simulink model "c00007M_harness"  (R2018a)
settings: Solver=ode3  StartTime=0.0  StopTime=10.0  RelTol=1e-3  EnableMultiTasking=on
undefined symbols (not defined in the file): b, DiscIntNeverNeededParam, J, K, L, PosMinimaW3, PosMinimaW4, R, sigbuilder_block
(part 13 of 74)

== system c00007M_harness/M171 ==
  DW1 : Inport  OutMin=0  OutMax=4  OutDataTypeStr=int8
  DW2 : Inport  Port=2  OutMin=0  OutMax=4  OutDataTypeStr=int8
  DW3 : Inport  Port=3  OutMin=0  OutMax=4  OutDataTypeStr=int8
  P1W2 : Inport  Port=4  OutMin=0  OutMax=4  OutDataTypeStr=int8
  P2W3 : Inport  Port=5  OutMin=0  OutMax=4  OutDataTypeStr=int8
  P3W4 : Inport  Port=6  OutMin=0  OutMax=4  OutDataTypeStr=int8
  O1 : Inport  Port=7  OutDataTypeStr=boolean
  O2 : Inport  Port=8  OutDataTypeStr=boolean
  O3 : Inport  Port=9  OutDataTypeStr=boolean
  O4 : Inport  Port=10  OutDataTypeStr=boolean
  LD : Inport  Port=11  OutDataTypeStr=boolean
  CW1C : Inport  Port=12  OutMin=0  OutMax=4  OutDataTypeStr=int8
  CW2C : Inport  Port=13  OutMin=0  OutMax=4  OutDataTypeStr=int8
  CW4C : Inport  Port=14  OutMin=0  OutMax=4  OutDataTypeStr=int8
  Cyber : Subsystem
  M{,1..3} (4 alike) : Memory
  Physical : Subsystem
  S1 : Subsystem
  S2 : Subsystem
  S3 : Subsystem
  S4 : Subsystem
  W1Pos : Outport
  W2Pos : Outport  Port=2
  W3Pos : Outport  Port=3
  W4Pos : Outport  Port=4
  wires:
  Cyber/4(W4) -> Physical/4(InW4)
  Physical/4(W4) -> S4/1(PhyMeasure), W4Pos/1
  DW2/1 -> Cyber/6(DW2)
  P3W4/1 -> Cyber/10(P3W4)
  S2/1(SensorOut) -> M1/1
  Physical/2(W2) -> S2/1(PhyMeasure), W2Pos/1
  DW1/1 -> Cyber/5(DW1)
  M/1 -> Cyber/1(PosW1)
  Physical/3(W3) -> S3/1(PhyMeasure), W3Pos/1
  M1/1 -> Cyber/2(PosW2)
  S4/1(SensorOut) -> M3/1
  DW3/1 -> Cyber/7(DW3)
  O3/1 -> Cyber/13(OW3)
  CW1C/1 -> Cyber/16(CW1C)
  P1W2/1 -> Cyber/8(P1W2)
  M2/1 -> Cyber/3(PosW3)
  Cyber/2(W2) -> Physical/2(InW2)
  Cyber/1(W1) -> Physical/1(InW1)
  O1/1 -> Cyber/11(OW1)
  LD/1 -> Cyber/15(LD)
  Cyber/3(W3) -> Physical/3(InW3)
  O2/1 -> Cyber/12(OW2)
  S3/1(SensorOut) -> M2/1
  O4/1 -> Cyber/14(OW4)
  Physical/1(W1) -> S1/1(PhyMeasure), W1Pos/1
  CW4C/1 -> Cyber/18(CW4C)
  CW2C/1 -> Cyber/17(CW2C)
  S1/1(SensorOut) -> M/1
  P2W3/1 -> Cyber/9(P2W3)
  M3/1 -> Cyber/4(PosW4)

== system c00007M_harness/M172 ==
  DW1 : Inport  OutMin=0  OutMax=4  OutDataTypeStr=int8
  DW2 : Inport  Port=2  OutMin=0  OutMax=4  OutDataTypeStr=int8
  DW3 : Inport  Port=3  OutMin=0  OutMax=4  OutDataTypeStr=int8
  P1W2 : Inport  Port=4  OutMin=0  OutMax=4  OutDataTypeStr=int8
  P2W3 : Inport  Port=5  OutMin=0  OutMax=4  OutDataTypeStr=int8
  P3W4 : Inport  Port=6  OutMin=0  OutMax=4  OutDataTypeStr=int8
  O1 : Inport  Port=7  OutDataTypeStr=boolean
  O2 : Inport  Port=8  OutDataTypeStr=boolean
  O3 : Inport  Port=9  OutDataTypeStr=boolean
  O4 : Inport  Port=10  OutDataTypeStr=boolean
  LD : Inport  Port=11  OutDataTypeStr=boolean
  CW1C : Inport  Port=12  OutMin=0  OutMax=4  OutDataTypeStr=int8
  CW2C : Inport  Port=13  OutMin=0  OutMax=4  OutDataTypeStr=int8
  CW4C : Inport  Port=14  OutMin=0  OutMax=4  OutDataTypeStr=int8
  Cyber : Subsystem
  M{,1..3} (4 alike) : Memory
  Physical : Subsystem
  S1 : Subsystem
  S2 : Subsystem
  S3 : Subsystem
  S4 : Subsystem
  W1Pos : Outport
  W2Pos : Outport  Port=2
  W3Pos : Outport  Port=3
  W4Pos : Outport  Port=4
  wires:
  Cyber/4(W4) -> Physical/4(InW4)
  Physical/4(W4) -> S4/1(PhyMeasure), W4Pos/1
  DW2/1 -> Cyber/6(DW2)
  P3W4/1 -> Cyber/10(P3W4)
  S2/1(SensorOut) -> M1/1
  Physical/2(W2) -> S2/1(PhyMeasure), W2Pos/1
  DW1/1 -> Cyber/5(DW1)
  M/1 -> Cyber/1(PosW1)
  Physical/3(W3) -> S3/1(PhyMeasure), W3Pos/1
  M1/1 -> Cyber/2(PosW2)
  S4/1(SensorOut) -> M3/1
  DW3/1 -> Cyber/7(DW3)
  O3/1 -> Cyber/13(OW3)
  CW1C/1 -> Cyber/16(CW1C)
  P1W2/1 -> Cyber/8(P1W2)
  M2/1 -> Cyber/3(PosW3)
  Cyber/2(W2) -> Physical/2(InW2)
  Cyber/1(W1) -> Physical/1(InW1)
  O1/1 -> Cyber/11(OW1)
  LD/1 -> Cyber/15(LD)
  Cyber/3(W3) -> Physical/3(InW3)
  O2/1 -> Cyber/12(OW2)
  S3/1(SensorOut) -> M2/1
  O4/1 -> Cyber/14(OW4)
  Physical/1(W1) -> S1/1(PhyMeasure), W1Pos/1
  CW4C/1 -> Cyber/18(CW4C)
  CW2C/1 -> Cyber/17(CW2C)
  S1/1(SensorOut) -> M/1
  P2W3/1 -> Cyber/9(P2W3)
  M3/1 -> Cyber/4(PosW4)

== system c00007M_harness/M173 ==
  DW1 : Inport  OutMin=0  OutMax=4  OutDataTypeStr=int8
  DW2 : Inport  Port=2  OutMin=0  OutMax=4  OutDataTypeStr=int8
  DW3 : Inport  Port=3  OutMin=0  OutMax=4  OutDataTypeStr=int8
  P1W2 : Inport  Port=4  OutMin=0  OutMax=4  OutDataTypeStr=int8
  P2W3 : Inport  Port=5  OutMin=0  OutMax=4  OutDataTypeStr=int8
  P3W4 : Inport  Port=6  OutMin=0  OutMax=4  OutDataTypeStr=int8
  O1 : Inport  Port=7  OutDataTypeStr=boolean
  O2 : Inport  Port=8  OutDataTypeStr=boolean
  O3 : Inport  Port=9  OutDataTypeStr=boolean
  O4 : Inport  Port=10  OutDataTypeStr=boolean
  LD : Inport  Port=11  OutDataTypeStr=boolean
  CW1C : Inport  Port=12  OutMin=0  OutMax=4  OutDataTypeStr=int8
  CW2C : Inport  Port=13  OutMin=0  OutMax=4  OutDataTypeStr=int8
  CW4C : Inport  Port=14  OutMin=0  OutMax=4  OutDataTypeStr=int8
  Cyber : Subsystem
  M{,1..3} (4 alike) : Memory
  Physical : Subsystem
  S1 : Subsystem
  S2 : Subsystem
  S3 : Subsystem
  S4 : Subsystem
  W1Pos : Outport
  W2Pos : Outport  Port=2
  W3Pos : Outport  Port=3
  W4Pos : Outport  Port=4
  wires:
  Cyber/4(W4) -> Physical/4(InW4)
  Physical/4(W4) -> S4/1(PhyMeasure), W4Pos/1
  DW2/1 -> Cyber/6(DW2)
  P3W4/1 -> Cyber/10(P3W4)
  S2/1(SensorOut) -> M1/1
  Physical/2(W2) -> S2/1(PhyMeasure), W2Pos/1
  DW1/1 -> Cyber/5(DW1)
  M/1 -> Cyber/1(PosW1)
  Physical/3(W3) -> S3/1(PhyMeasure), W3Pos/1
  M1/1 -> Cyber/2(PosW2)
  S4/1(SensorOut) -> M3/1
  DW3/1 -> Cyber/7(DW3)
  O3/1 -> Cyber/13(OW3)
  CW1C/1 -> Cyber/16(CW1C)
  P1W2/1 -> Cyber/8(P1W2)
  M2/1 -> Cyber/3(PosW3)
  Cyber/2(W2) -> Physical/2(InW2)
  Cyber/1(W1) -> Physical/1(InW1)
  O1/1 -> Cyber/11(OW1)
  LD/1 -> Cyber/15(LD)
  Cyber/3(W3) -> Physical/3(InW3)
  O2/1 -> Cyber/12(OW2)
  S3/1(SensorOut) -> M2/1
  O4/1 -> Cyber/14(OW4)
  Physical/1(W1) -> S1/1(PhyMeasure), W1Pos/1
  CW4C/1 -> Cyber/18(CW4C)
  CW2C/1 -> Cyber/17(CW2C)
  S1/1(SensorOut) -> M/1
  P2W3/1 -> Cyber/9(P2W3)
  M3/1 -> Cyber/4(PosW4)

== system c00007M_harness/M174 ==
  DW1 : Inport  OutMin=0  OutMax=4  OutDataTypeStr=int8
  DW2 : Inport  Port=2  OutMin=0  OutMax=4  OutDataTypeStr=int8
  DW3 : Inport  Port=3  OutMin=0  OutMax=4  OutDataTypeStr=int8
  P1W2 : Inport  Port=4  OutMin=0  OutMax=4  OutDataTypeStr=int8
  P2W3 : Inport  Port=5  OutMin=0  OutMax=4  OutDataTypeStr=int8
  P3W4 : Inport  Port=6  OutMin=0  OutMax=4  OutDataTypeStr=int8
  O1 : Inport  Port=7  OutDataTypeStr=boolean
  O2 : Inport  Port=8  OutDataTypeStr=boolean
  O3 : Inport  Port=9  OutDataTypeStr=boolean
  O4 : Inport  Port=10  OutDataTypeStr=boolean
  LD : Inport  Port=11  OutDataTypeStr=boolean
  CW1C : Inport  Port=12  OutMin=0  OutMax=4  OutDataTypeStr=int8
  CW2C : Inport  Port=13  OutMin=0  OutMax=4  OutDataTypeStr=int8
  CW4C : Inport  Port=14  OutMin=0  OutMax=4  OutDataTypeStr=int8
  Cyber : Subsystem
  M{,1..3} (4 alike) : Memory
  Physical : Subsystem
  S1 : Subsystem
  S2 : Subsystem
  S3 : Subsystem
  S4 : Subsystem
  W1Pos : Outport
  W2Pos : Outport  Port=2
  W3Pos : Outport  Port=3
  W4Pos : Outport  Port=4
  wires:
  Cyber/4(W4) -> Physical/4(InW4)
  Physical/4(W4) -> S4/1(PhyMeasure), W4Pos/1
  DW2/1 -> Cyber/6(DW2)
  P3W4/1 -> Cyber/10(P3W4)
  S2/1(SensorOut) -> M1/1
  Physical/2(W2) -> S2/1(PhyMeasure), W2Pos/1
  DW1/1 -> Cyber/5(DW1)
  M/1 -> Cyber/1(PosW1)
  Physical/3(W3) -> S3/1(PhyMeasure), W3Pos/1
  M1/1 -> Cyber/2(PosW2)
  S4/1(SensorOut) -> M3/1
  DW3/1 -> Cyber/7(DW3)
  O3/1 -> Cyber/13(OW3)
  CW1C/1 -> Cyber/16(CW1C)
  P1W2/1 -> Cyber/8(P1W2)
  M2/1 -> Cyber/3(PosW3)
  Cyber/2(W2) -> Physical/2(InW2)
  Cyber/1(W1) -> Physical/1(InW1)
  O1/1 -> Cyber/11(OW1)
  LD/1 -> Cyber/15(LD)
  Cyber/3(W3) -> Physical/3(InW3)
  O2/1 -> Cyber/12(OW2)
  S3/1(SensorOut) -> M2/1
  O4/1 -> Cyber/14(OW4)
  Physical/1(W1) -> S1/1(PhyMeasure), W1Pos/1
  CW4C/1 -> Cyber/18(CW4C)
  CW2C/1 -> Cyber/17(CW2C)
  S1/1(SensorOut) -> M/1
  P2W3/1 -> Cyber/9(P2W3)
  M3/1 -> Cyber/4(PosW4)

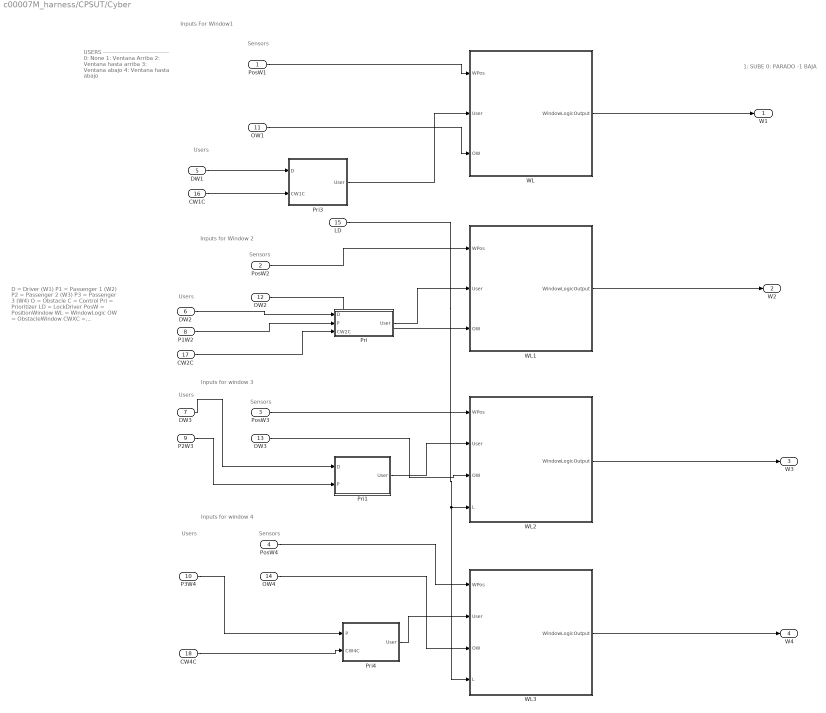
== system c00007M_harness/CPSUT/Cyber ==
  note: D = Driver (W1)
      | P1 = Passenger 1 (W2)
      | P2 = Passenger 2 (W3)
      | P3 = Passenger 3 (W4)
      | O = Obstacle
      | C = Control
      | Pri = Prioritizer
      | LD = LockDriver
      | PosW = PositionWindow
      | WL = WindowLogic
      | OW = ObstacleWindow
      | CWXC = ControlWindowXCentralized
      | S = Sensor
      | L = Lock
      | WPos = WindowPosition
      | M = Memory
      | InW = InputWindow
      | WIn = WindowInput
  note: 1: SUBE
      | 0: PARADO
      | -1 BAJA
  note: USERS
      | ---------------------------------
      | 0: None
      | 1: Ventana Arriba
      | 2: Ventana hasta arriba
      | 3: Ventana abajo
      | 4: Ventana hasta abajo
  note: Sensors
  note: Users
  note: Sensors
  note: Users
  note: Sensors
  note: Users
  note: Users
  note: Inputs for window 4
  note: Inputs for window 3
  note: Inputs for Window 2
  note: Inputs For Window1
  note: Sensors
  PosW1 : Inport
  PosW2 : Inport  Port=2
  PosW3 : Inport  Port=3
  PosW4 : Inport  Port=4
  DW1 : Inport  Port=5
  DW2 : Inport  Port=6
  DW3 : Inport  Port=7
  P1W2 : Inport  Port=8
  P2W3 : Inport  Port=9
  P3W4 : Inport  Port=10
  OW1 : Inport  Port=11
  OW2 : Inport  Port=12
  OW3 : Inport  Port=13
  OW4 : Inport  Port=14
  LD : Inport  Port=15
  CW1C : Inport  Port=16
  CW2C : Inport  Port=17
  CW4C : Inport  Port=18
  Pri : Subsystem
  Pri1 : Subsystem
  Pri3 : Subsystem
  Pri4 : Subsystem
  WL : Subsystem
  WL1 : Subsystem
  WL2 : Subsystem
  WL3 : Subsystem
  W1 : Outport
  W2 : Outport  Port=2
  W3 : Outport  Port=3
  W4 : Outport  Port=4
  wires:
  LD/1 -> WL3/4(L), WL2/4(L)
  PosW1/1 -> WL/1(WPos)
  OW1/1 -> WL/3(OW)
  DW1/1 -> Pri3/1(D)
  WL/1(WindowLogicOutput) -> W1/1
  Pri/1(User) -> WL1/2(User)
  DW2/1 -> Pri/1(D)
  P1W2/1 -> Pri/2(P)
  PosW2/1 -> WL1/1(WPos)
  OW2/1 -> WL1/3(OW)
  WL1/1(WindowLogicOutput) -> W2/1
  Pri1/1(User) -> WL2/2(User)
  PosW3/1 -> WL2/1(WPos)
  OW3/1 -> WL2/3(OW)
  DW3/1 -> Pri1/1(D)
  P2W3/1 -> Pri1/2(P)
  P3W4/1 -> Pri4/1(P)
  PosW4/1 -> WL3/1(WPos)
  OW4/1 -> WL3/3(OW)
  Pri4/1(User) -> WL3/2(User)
  WL2/1(WindowLogicOutput) -> W3/1
  WL3/1(WindowLogicOutput) -> W4/1
  Pri3/1(User) -> WL/2(User)
  CW1C/1 -> Pri3/2(CW1C)
  CW2C/1 -> Pri/3(CW2C)
  CW4C/1 -> Pri4/2(CW4C)

== system c00007M_harness/CPSUT/Physical ==
  InW1 : Inport
  InW2 : Inport  Port=2
  InW3 : Inport  Port=3
  InW4 : Inport  Port=4
  W : Subsystem
  W5 : Subsystem
  W6 : Subsystem
  W7 : Subsystem
  W1 : Outport
  W2 : Outport  Port=2
  W3 : Outport  Port=3
  W4 : Outport  Port=4
  wires:
  InW1/1 -> W/1(WIn)
  InW2/1 -> W5/1(WIn)
  InW3/1 -> W6/1(WIn)
  InW4/1 -> W7/1(WIn)
  W/1(WPos) -> W1/1
  W5/1(WPos) -> W2/1
  W6/1(WPos) -> W3/1
  W7/1(WPos) -> W4/1

== system c00007M_harness/CPSUT/S1 ==
  PhyMeasure : Inport
  SensorOut : Outport
  wires:
  PhyMeasure/1 -> SensorOut/1

== system c00007M_harness/CPSUT/S2 ==
  PhyMeasure : Inport
  SensorOut : Outport
  wires:
  PhyMeasure/1 -> SensorOut/1

== system c00007M_harness/CPSUT/S3 ==
  PhyMeasure : Inport
  SensorOut : Outport
  wires:
  PhyMeasure/1 -> SensorOut/1

== system c00007M_harness/CPSUT/S4 ==
  PhyMeasure : Inport
  SensorOut : Outport
  wires:
  PhyMeasure/1 -> SensorOut/1

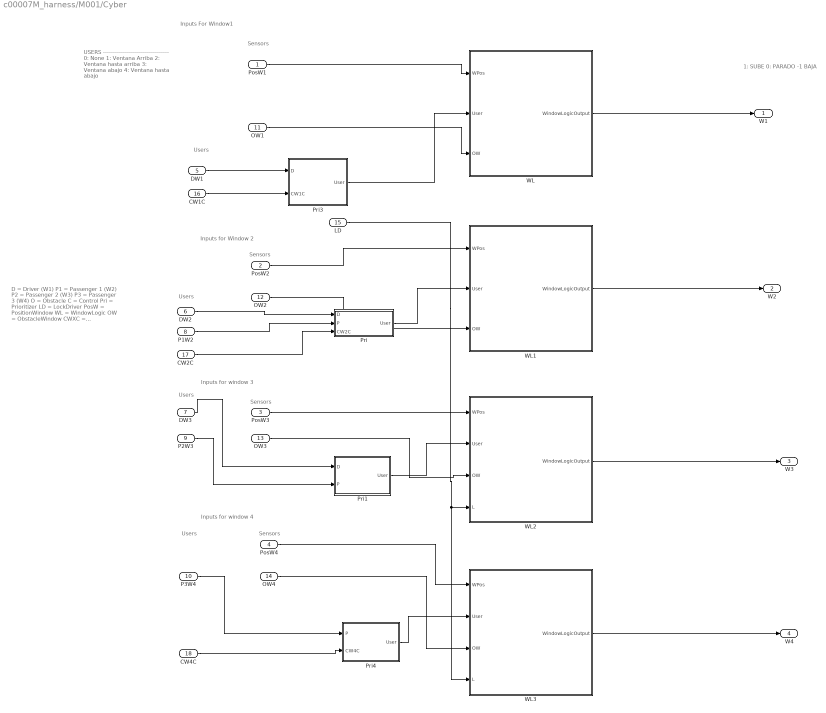
== system c00007M_harness/M001/Cyber ==
  note: D = Driver (W1)
      | P1 = Passenger 1 (W2)
      | P2 = Passenger 2 (W3)
      | P3 = Passenger 3 (W4)
      | O = Obstacle
      | C = Control
      | Pri = Prioritizer
      | LD = LockDriver
      | PosW = PositionWindow
      | WL = WindowLogic
      | OW = ObstacleWindow
      | CWXC = ControlWindowXCentralized
      | S = Sensor
      | L = Lock
      | WPos = WindowPosition
      | M = Memory
      | InW = InputWindow
      | WIn = WindowInput
  note: 1: SUBE
      | 0: PARADO
      | -1 BAJA
  note: USERS
      | ---------------------------------
      | 0: None
      | 1: Ventana Arriba
      | 2: Ventana hasta arriba
      | 3: Ventana abajo
      | 4: Ventana hasta abajo
  note: Sensors
  note: Users
  note: Sensors
  note: Users
  note: Sensors
  note: Users
  note: Users
  note: Inputs for window 4
  note: Inputs for window 3
  note: Inputs for Window 2
  note: Inputs For Window1
  note: Sensors
  PosW1 : Inport
  PosW2 : Inport  Port=2
  PosW3 : Inport  Port=3
  PosW4 : Inport  Port=4
  DW1 : Inport  Port=5
  DW2 : Inport  Port=6
  DW3 : Inport  Port=7
  P1W2 : Inport  Port=8
  P2W3 : Inport  Port=9
  P3W4 : Inport  Port=10
  OW1 : Inport  Port=11
  OW2 : Inport  Port=12
  OW3 : Inport  Port=13
  OW4 : Inport  Port=14
  LD : Inport  Port=15
  CW1C : Inport  Port=16
  CW2C : Inport  Port=17
  CW4C : Inport  Port=18
  Pri : Subsystem
  Pri1 : Subsystem
  Pri3 : Subsystem
  Pri4 : Subsystem
  WL : Subsystem
  WL1 : Subsystem
  WL2 : Subsystem
  WL3 : Subsystem
  W1 : Outport
  W2 : Outport  Port=2
  W3 : Outport  Port=3
  W4 : Outport  Port=4
  wires:
  LD/1 -> WL3/4(L), WL2/4(L)
  PosW1/1 -> WL/1(WPos)
  OW1/1 -> WL/3(OW)
  DW1/1 -> Pri3/1(D)
  WL/1(WindowLogicOutput) -> W1/1
  Pri/1(User) -> WL1/2(User)
  DW2/1 -> Pri/1(D)
  P1W2/1 -> Pri/2(P)
  PosW2/1 -> WL1/1(WPos)
  OW2/1 -> WL1/3(OW)
  WL1/1(WindowLogicOutput) -> W2/1
  Pri1/1(User) -> WL2/2(User)
  PosW3/1 -> WL2/1(WPos)
  OW3/1 -> WL2/3(OW)
  DW3/1 -> Pri1/1(D)
  P2W3/1 -> Pri1/2(P)
  P3W4/1 -> Pri4/1(P)
  PosW4/1 -> WL3/1(WPos)
  OW4/1 -> WL3/3(OW)
  Pri4/1(User) -> WL3/2(User)
  WL2/1(WindowLogicOutput) -> W3/1
  WL3/1(WindowLogicOutput) -> W4/1
  Pri3/1(User) -> WL/2(User)
  CW1C/1 -> Pri3/2(CW1C)
  CW2C/1 -> Pri/3(CW2C)
  CW4C/1 -> Pri4/2(CW4C)

== system c00007M_harness/M001/Physical ==
  InW1 : Inport
  InW2 : Inport  Port=2
  InW3 : Inport  Port=3
  InW4 : Inport  Port=4
  W : Subsystem
  W5 : Subsystem
  W6 : Subsystem
  W7 : Subsystem
  W1 : Outport
  W2 : Outport  Port=2
  W3 : Outport  Port=3
  W4 : Outport  Port=4
  wires:
  InW1/1 -> W/1(WIn)
  InW2/1 -> W5/1(WIn)
  InW3/1 -> W6/1(WIn)
  InW4/1 -> W7/1(WIn)
  W/1(WPos) -> W1/1
  W5/1(WPos) -> W2/1
  W6/1(WPos) -> W3/1
  W7/1(WPos) -> W4/1

== system c00007M_harness/M001/S1 ==
  PhyMeasure : Inport
  SensorOut : Outport
  wires:
  PhyMeasure/1 -> SensorOut/1

== system c00007M_harness/M001/S2 ==
  PhyMeasure : Inport
  SensorOut : Outport
  wires:
  PhyMeasure/1 -> SensorOut/1

== system c00007M_harness/M001/S3 ==
  PhyMeasure : Inport
  SensorOut : Outport
  wires:
  PhyMeasure/1 -> SensorOut/1

== system c00007M_harness/M001/S4 ==
  PhyMeasure : Inport
  SensorOut : Outport
  wires:
  PhyMeasure/1 -> SensorOut/1

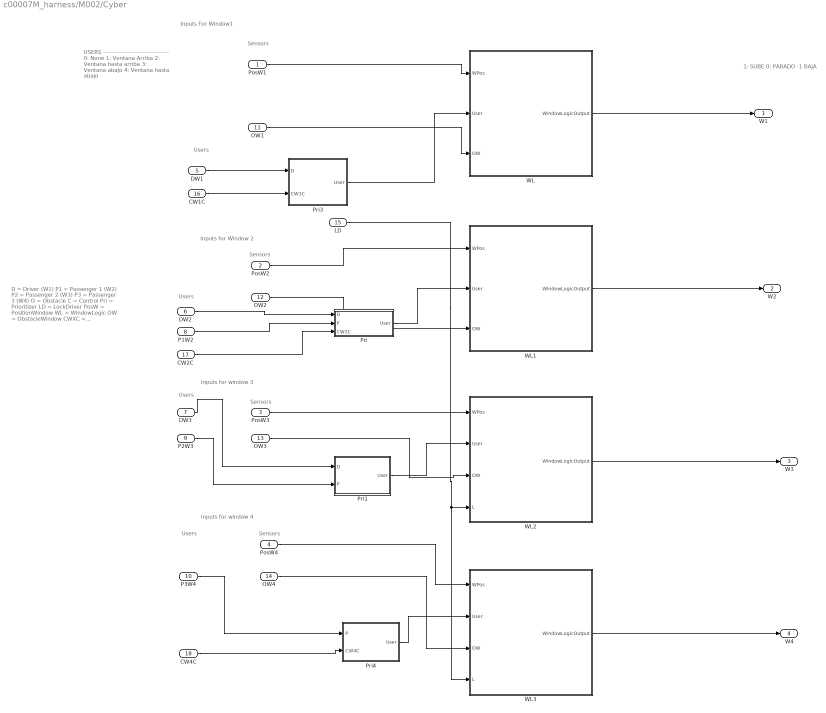
== system c00007M_harness/M002/Cyber ==
  note: Sensors
  note: Inputs For Window1
  note: Inputs for Window 2
  note: Inputs for window 3
  note: Inputs for window 4
  note: Users
  note: Users
  note: Sensors
  note: Users
  note: Sensors
  note: Users
  note: Sensors
  note: USERS
      | ---------------------------------
      | 0: None
      | 1: Ventana Arriba
      | 2: Ventana hasta arriba
      | 3: Ventana abajo
      | 4: Ventana hasta abajo
  note: 1: SUBE
      | 0: PARADO
      | -1 BAJA
  note: D = Driver (W1)
      | P1 = Passenger 1 (W2)
      | P2 = Passenger 2 (W3)
      | P3 = Passenger 3 (W4)
      | O = Obstacle
      | C = Control
      | Pri = Prioritizer
      | LD = LockDriver
      | PosW = PositionWindow
      | WL = WindowLogic
      | OW = ObstacleWindow
      | CWXC = ControlWindowXCentralized
      | S = Sensor
      | L = Lock
      | WPos = WindowPosition
      | M = Memory
      | InW = InputWindow
      | WIn = WindowInput
  PosW1 : Inport
  PosW2 : Inport  Port=2
  PosW3 : Inport  Port=3
  PosW4 : Inport  Port=4
  DW1 : Inport  Port=5
  DW2 : Inport  Port=6
  DW3 : Inport  Port=7
  P1W2 : Inport  Port=8
  P2W3 : Inport  Port=9
  P3W4 : Inport  Port=10
  OW1 : Inport  Port=11
  OW2 : Inport  Port=12
  OW3 : Inport  Port=13
  OW4 : Inport  Port=14
  LD : Inport  Port=15
  CW1C : Inport  Port=16
  CW2C : Inport  Port=17
  CW4C : Inport  Port=18
  Pri : Subsystem
  Pri1 : Subsystem
  Pri3 : Subsystem
  Pri4 : Subsystem
  WL : Subsystem
  WL1 : Subsystem
  WL2 : Subsystem
  WL3 : Subsystem
  W1 : Outport
  W2 : Outport  Port=2
  W3 : Outport  Port=3
  W4 : Outport  Port=4
  wires:
  CW4C/1 -> Pri4/2(CW4C)
  CW2C/1 -> Pri/3(CW2C)
  CW1C/1 -> Pri3/2(CW1C)
  Pri3/1(User) -> WL/2(User)
  WL3/1(WindowLogicOutput) -> W4/1
  WL2/1(WindowLogicOutput) -> W3/1
  Pri4/1(User) -> WL3/2(User)
  OW4/1 -> WL3/3(OW)
  PosW4/1 -> WL3/1(WPos)
  P3W4/1 -> Pri4/1(P)
  P2W3/1 -> Pri1/2(P)
  DW3/1 -> Pri1/1(D)
  OW3/1 -> WL2/3(OW)
  PosW3/1 -> WL2/1(WPos)
  Pri1/1(User) -> WL2/2(User)
  WL1/1(WindowLogicOutput) -> W2/1
  OW2/1 -> WL1/3(OW)
  PosW2/1 -> WL1/1(WPos)
  P1W2/1 -> Pri/2(P)
  DW2/1 -> Pri/1(D)
  Pri/1(User) -> WL1/2(User)
  WL/1(WindowLogicOutput) -> W1/1
  DW1/1 -> Pri3/1(D)
  OW1/1 -> WL/3(OW)
  PosW1/1 -> WL/1(WPos)
  LD/1 -> WL2/4(L), WL3/4(L)

== system c00007M_harness/M002/Physical ==
  InW1 : Inport
  InW2 : Inport  Port=2
  InW3 : Inport  Port=3
  InW4 : Inport  Port=4
  W : Subsystem
  W5 : Subsystem
  W6 : Subsystem
  W7 : Subsystem
  W1 : Outport
  W2 : Outport  Port=2
  W3 : Outport  Port=3
  W4 : Outport  Port=4
  wires:
  W7/1(WPos) -> W4/1
  W6/1(WPos) -> W3/1
  W5/1(WPos) -> W2/1
  W/1(WPos) -> W1/1
  InW4/1 -> W7/1(WIn)
  InW3/1 -> W6/1(WIn)
  InW2/1 -> W5/1(WIn)
  InW1/1 -> W/1(WIn)

== system c00007M_harness/M002/S1 ==
  PhyMeasure : Inport
  SensorOut : Outport
  wires:
  PhyMeasure/1 -> SensorOut/1

== system c00007M_harness/M002/S2 ==
  PhyMeasure : Inport
  SensorOut : Outport
  wires:
  PhyMeasure/1 -> SensorOut/1

== system c00007M_harness/M002/S3 ==
  PhyMeasure : Inport
  SensorOut : Outport
  wires:
  PhyMeasure/1 -> SensorOut/1

== system c00007M_harness/M002/S4 ==
  PhyMeasure : Inport
  SensorOut : Outport
  wires:
  PhyMeasure/1 -> SensorOut/1

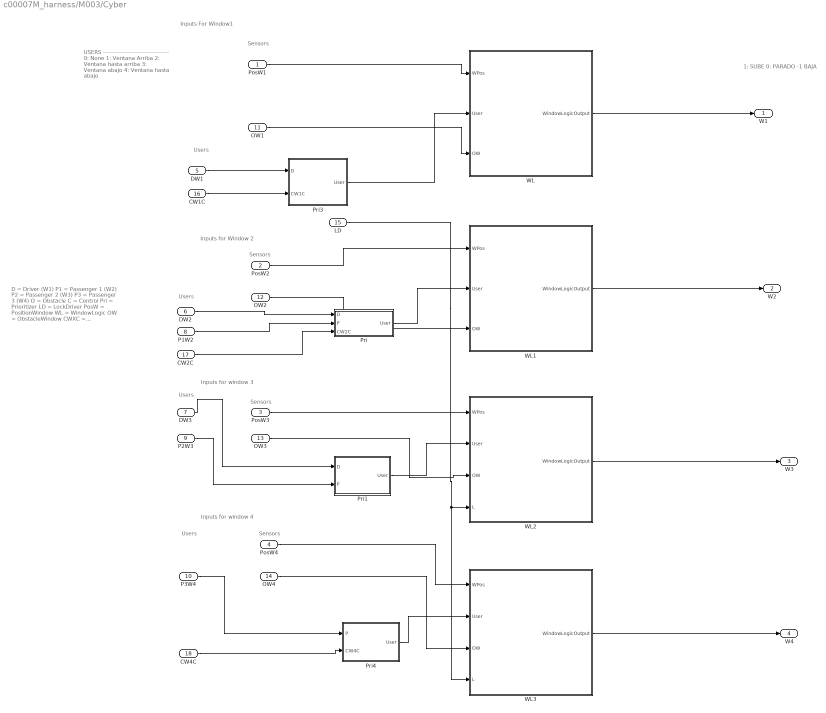
== system c00007M_harness/M003/Cyber ==
  note: Sensors
  note: Inputs For Window1
  note: Inputs for Window 2
  note: Inputs for window 3
  note: Inputs for window 4
  note: Users
  note: Users
  note: Sensors
  note: Users
  note: Sensors
  note: Users
  note: Sensors
  note: USERS
      | ---------------------------------
      | 0: None
      | 1: Ventana Arriba
      | 2: Ventana hasta arriba
      | 3: Ventana abajo
      | 4: Ventana hasta abajo
  note: 1: SUBE
      | 0: PARADO
      | -1 BAJA
  note: D = Driver (W1)
      | P1 = Passenger 1 (W2)
      | P2 = Passenger 2 (W3)
      | P3 = Passenger 3 (W4)
      | O = Obstacle
      | C = Control
      | Pri = Prioritizer
      | LD = LockDriver
      | PosW = PositionWindow
      | WL = WindowLogic
      | OW = ObstacleWindow
      | CWXC = ControlWindowXCentralized
      | S = Sensor
      | L = Lock
      | WPos = WindowPosition
      | M = Memory
      | InW = InputWindow
      | WIn = WindowInput
  PosW1 : Inport
  PosW2 : Inport  Port=2
  PosW3 : Inport  Port=3
  PosW4 : Inport  Port=4
  DW1 : Inport  Port=5
  DW2 : Inport  Port=6
  DW3 : Inport  Port=7
  P1W2 : Inport  Port=8
  P2W3 : Inport  Port=9
  P3W4 : Inport  Port=10
  OW1 : Inport  Port=11
  OW2 : Inport  Port=12
  OW3 : Inport  Port=13
  OW4 : Inport  Port=14
  LD : Inport  Port=15
  CW1C : Inport  Port=16
  CW2C : Inport  Port=17
  CW4C : Inport  Port=18
  Pri : Subsystem
  Pri1 : Subsystem
  Pri3 : Subsystem
  Pri4 : Subsystem
  WL : Subsystem
  WL1 : Subsystem
  WL2 : Subsystem
  WL3 : Subsystem
  W1 : Outport
  W2 : Outport  Port=2
  W3 : Outport  Port=3
  W4 : Outport  Port=4
  wires:
  CW4C/1 -> Pri4/2(CW4C)
  CW2C/1 -> Pri/3(CW2C)
  CW1C/1 -> Pri3/2(CW1C)
  Pri3/1(User) -> WL/2(User)
  WL3/1(WindowLogicOutput) -> W4/1
  WL2/1(WindowLogicOutput) -> W3/1
  Pri4/1(User) -> WL3/2(User)
  OW4/1 -> WL3/3(OW)
  PosW4/1 -> WL3/1(WPos)
  P3W4/1 -> Pri4/1(P)
  P2W3/1 -> Pri1/2(P)
  DW3/1 -> Pri1/1(D)
  OW3/1 -> WL2/3(OW)
  PosW3/1 -> WL2/1(WPos)
  Pri1/1(User) -> WL2/2(User)
  WL1/1(WindowLogicOutput) -> W2/1
  OW2/1 -> WL1/3(OW)
  PosW2/1 -> WL1/1(WPos)
  P1W2/1 -> Pri/2(P)
  DW2/1 -> Pri/1(D)
  Pri/1(User) -> WL1/2(User)
  WL/1(WindowLogicOutput) -> W1/1
  DW1/1 -> Pri3/1(D)
  OW1/1 -> WL/3(OW)
  PosW1/1 -> WL/1(WPos)
  LD/1 -> WL2/4(L), WL3/4(L)

== system c00007M_harness/M003/Physical ==
  InW1 : Inport
  InW2 : Inport  Port=2
  InW3 : Inport  Port=3
  InW4 : Inport  Port=4
  W : Subsystem
  W5 : Subsystem
  W6 : Subsystem
  W7 : Subsystem
  W1 : Outport
  W2 : Outport  Port=2
  W3 : Outport  Port=3
  W4 : Outport  Port=4
  wires:
  W7/1(WPos) -> W4/1
  W6/1(WPos) -> W3/1
  W5/1(WPos) -> W2/1
  W/1(WPos) -> W1/1
  InW4/1 -> W7/1(WIn)
  InW3/1 -> W6/1(WIn)
  InW2/1 -> W5/1(WIn)
  InW1/1 -> W/1(WIn)

== system c00007M_harness/M003/S1 ==
  PhyMeasure : Inport
  SensorOut : Outport
  wires:
  PhyMeasure/1 -> SensorOut/1

== system c00007M_harness/M003/S2 ==
  PhyMeasure : Inport
  SensorOut : Outport
  wires:
  PhyMeasure/1 -> SensorOut/1

== system c00007M_harness/M003/S3 ==
  PhyMeasure : Inport
  SensorOut : Outport
  wires:
  PhyMeasure/1 -> SensorOut/1

== system c00007M_harness/M003/S4 ==
  PhyMeasure : Inport
  SensorOut : Outport
  wires:
  PhyMeasure/1 -> SensorOut/1

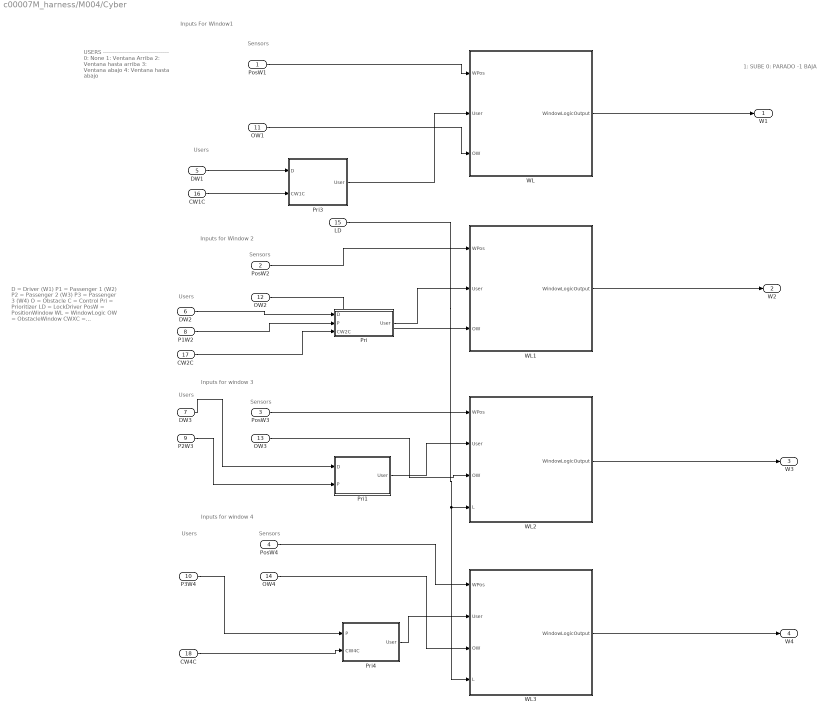
== system c00007M_harness/M004/Cyber ==
  note: Sensors
  note: Inputs For Window1
  note: Inputs for Window 2
  note: Inputs for window 3
  note: Inputs for window 4
  note: Users
  note: Users
  note: Sensors
  note: Users
  note: Sensors
  note: Users
  note: Sensors
  note: USERS
      | ---------------------------------
      | 0: None
      | 1: Ventana Arriba
      | 2: Ventana hasta arriba
      | 3: Ventana abajo
      | 4: Ventana hasta abajo
  note: 1: SUBE
      | 0: PARADO
      | -1 BAJA
  note: D = Driver (W1)
      | P1 = Passenger 1 (W2)
      | P2 = Passenger 2 (W3)
      | P3 = Passenger 3 (W4)
      | O = Obstacle
      | C = Control
      | Pri = Prioritizer
      | LD = LockDriver
      | PosW = PositionWindow
      | WL = WindowLogic
      | OW = ObstacleWindow
      | CWXC = ControlWindowXCentralized
      | S = Sensor
      | L = Lock
      | WPos = WindowPosition
      | M = Memory
      | InW = InputWindow
      | WIn = WindowInput
  PosW1 : Inport
  PosW2 : Inport  Port=2
  PosW3 : Inport  Port=3
  PosW4 : Inport  Port=4
  DW1 : Inport  Port=5
  DW2 : Inport  Port=6
  DW3 : Inport  Port=7
  P1W2 : Inport  Port=8
  P2W3 : Inport  Port=9
  P3W4 : Inport  Port=10
  OW1 : Inport  Port=11
  OW2 : Inport  Port=12
  OW3 : Inport  Port=13
  OW4 : Inport  Port=14
  LD : Inport  Port=15
  CW1C : Inport  Port=16
  CW2C : Inport  Port=17
  CW4C : Inport  Port=18
  Pri : Subsystem
  Pri1 : Subsystem
  Pri3 : Subsystem
  Pri4 : Subsystem
  WL : Subsystem
  WL1 : Subsystem
  WL2 : Subsystem
  WL3 : Subsystem
  W1 : Outport
  W2 : Outport  Port=2
  W3 : Outport  Port=3
  W4 : Outport  Port=4
  wires:
  CW4C/1 -> Pri4/2(CW4C)
  CW2C/1 -> Pri/3(CW2C)
  CW1C/1 -> Pri3/2(CW1C)
  Pri3/1(User) -> WL/2(User)
  WL3/1(WindowLogicOutput) -> W4/1
  WL2/1(WindowLogicOutput) -> W3/1
  Pri4/1(User) -> WL3/2(User)
  OW4/1 -> WL3/3(OW)
  PosW4/1 -> WL3/1(WPos)
  P3W4/1 -> Pri4/1(P)
  P2W3/1 -> Pri1/2(P)
  DW3/1 -> Pri1/1(D)
  OW3/1 -> WL2/3(OW)
  PosW3/1 -> WL2/1(WPos)
  Pri1/1(User) -> WL2/2(User)
  WL1/1(WindowLogicOutput) -> W2/1
  OW2/1 -> WL1/3(OW)
  PosW2/1 -> WL1/1(WPos)
  P1W2/1 -> Pri/2(P)
  DW2/1 -> Pri/1(D)
  Pri/1(User) -> WL1/2(User)
  WL/1(WindowLogicOutput) -> W1/1
  DW1/1 -> Pri3/1(D)
  OW1/1 -> WL/3(OW)
  PosW1/1 -> WL/1(WPos)
  LD/1 -> WL2/4(L), WL3/4(L)

== system c00007M_harness/M004/Physical ==
  InW1 : Inport
  InW2 : Inport  Port=2
  InW3 : Inport  Port=3
  InW4 : Inport  Port=4
  W : Subsystem
  W5 : Subsystem
  W6 : Subsystem
  W7 : Subsystem
  W1 : Outport
  W2 : Outport  Port=2
  W3 : Outport  Port=3
  W4 : Outport  Port=4
  wires:
  W7/1(WPos) -> W4/1
  W6/1(WPos) -> W3/1
  W5/1(WPos) -> W2/1
  W/1(WPos) -> W1/1
  InW4/1 -> W7/1(WIn)
  InW3/1 -> W6/1(WIn)
  InW2/1 -> W5/1(WIn)
  InW1/1 -> W/1(WIn)

== system c00007M_harness/M004/S1 ==
  PhyMeasure : Inport
  SensorOut : Outport
  wires:
  PhyMeasure/1 -> SensorOut/1

== system c00007M_harness/M004/S2 ==
  PhyMeasure : Inport
  SensorOut : Outport
  wires:
  PhyMeasure/1 -> SensorOut/1

== system c00007M_harness/M004/S3 ==
  PhyMeasure : Inport
  SensorOut : Outport
  wires:
  PhyMeasure/1 -> SensorOut/1

== system c00007M_harness/M004/S4 ==
  PhyMeasure : Inport
  SensorOut : Outport
  wires:
  PhyMeasure/1 -> SensorOut/1

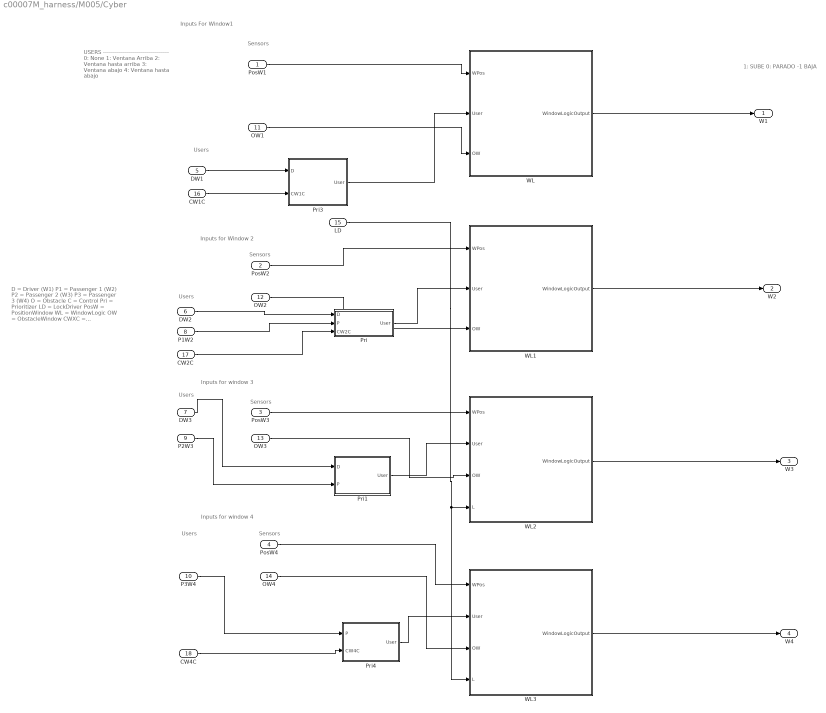
== system c00007M_harness/M005/Cyber ==
  note: Sensors
  note: Inputs For Window1
  note: Inputs for Window 2
  note: Inputs for window 3
  note: Inputs for window 4
  note: Users
  note: Users
  note: Sensors
  note: Users
  note: Sensors
  note: Users
  note: Sensors
  note: USERS
      | ---------------------------------
      | 0: None
      | 1: Ventana Arriba
      | 2: Ventana hasta arriba
      | 3: Ventana abajo
      | 4: Ventana hasta abajo
  note: 1: SUBE
      | 0: PARADO
      | -1 BAJA
  note: D = Driver (W1)
      | P1 = Passenger 1 (W2)
      | P2 = Passenger 2 (W3)
      | P3 = Passenger 3 (W4)
      | O = Obstacle
      | C = Control
      | Pri = Prioritizer
      | LD = LockDriver
      | PosW = PositionWindow
      | WL = WindowLogic
      | OW = ObstacleWindow
      | CWXC = ControlWindowXCentralized
      | S = Sensor
      | L = Lock
      | WPos = WindowPosition
      | M = Memory
      | InW = InputWindow
      | WIn = WindowInput
  PosW1 : Inport
  PosW2 : Inport  Port=2
  PosW3 : Inport  Port=3
  PosW4 : Inport  Port=4
  DW1 : Inport  Port=5
  DW2 : Inport  Port=6
  DW3 : Inport  Port=7
  P1W2 : Inport  Port=8
  P2W3 : Inport  Port=9
  P3W4 : Inport  Port=10
  OW1 : Inport  Port=11
  OW2 : Inport  Port=12
  OW3 : Inport  Port=13
  OW4 : Inport  Port=14
  LD : Inport  Port=15
  CW1C : Inport  Port=16
  CW2C : Inport  Port=17
  CW4C : Inport  Port=18
  Pri : Subsystem
  Pri1 : Subsystem
  Pri3 : Subsystem
  Pri4 : Subsystem
  WL : Subsystem
  WL1 : Subsystem
  WL2 : Subsystem
  WL3 : Subsystem
  W1 : Outport
  W2 : Outport  Port=2
  W3 : Outport  Port=3
  W4 : Outport  Port=4
  wires:
  CW4C/1 -> Pri4/2(CW4C)
  CW2C/1 -> Pri/3(CW2C)
  CW1C/1 -> Pri3/2(CW1C)
  Pri3/1(User) -> WL/2(User)
  WL3/1(WindowLogicOutput) -> W4/1
  WL2/1(WindowLogicOutput) -> W3/1
  Pri4/1(User) -> WL3/2(User)
  OW4/1 -> WL3/3(OW)
  PosW4/1 -> WL3/1(WPos)
  P3W4/1 -> Pri4/1(P)
  P2W3/1 -> Pri1/2(P)
  DW3/1 -> Pri1/1(D)
  OW3/1 -> WL2/3(OW)
  PosW3/1 -> WL2/1(WPos)
  Pri1/1(User) -> WL2/2(User)
  WL1/1(WindowLogicOutput) -> W2/1
  OW2/1 -> WL1/3(OW)
  PosW2/1 -> WL1/1(WPos)
  P1W2/1 -> Pri/2(P)
  DW2/1 -> Pri/1(D)
  Pri/1(User) -> WL1/2(User)
  WL/1(WindowLogicOutput) -> W1/1
  DW1/1 -> Pri3/1(D)
  OW1/1 -> WL/3(OW)
  PosW1/1 -> WL/1(WPos)
  LD/1 -> WL2/4(L), WL3/4(L)

== system c00007M_harness/M005/Physical ==
  InW1 : Inport
  InW2 : Inport  Port=2
  InW3 : Inport  Port=3
  InW4 : Inport  Port=4
  W : Subsystem
  W5 : Subsystem
  W6 : Subsystem
  W7 : Subsystem
  W1 : Outport
  W2 : Outport  Port=2
  W3 : Outport  Port=3
  W4 : Outport  Port=4
  wires:
  W7/1(WPos) -> W4/1
  W6/1(WPos) -> W3/1
  W5/1(WPos) -> W2/1
  W/1(WPos) -> W1/1
  InW4/1 -> W7/1(WIn)
  InW3/1 -> W6/1(WIn)
  InW2/1 -> W5/1(WIn)
  InW1/1 -> W/1(WIn)

== system c00007M_harness/M005/S1 ==
  PhyMeasure : Inport
  SensorOut : Outport
  wires:
  PhyMeasure/1 -> SensorOut/1

== system c00007M_harness/M005/S2 ==
  PhyMeasure : Inport
  SensorOut : Outport
  wires:
  PhyMeasure/1 -> SensorOut/1

== system c00007M_harness/M005/S3 ==
  PhyMeasure : Inport
  SensorOut : Outport
  wires:
  PhyMeasure/1 -> SensorOut/1

== system c00007M_harness/M005/S4 ==
  PhyMeasure : Inport
  SensorOut : Outport
  wires:
  PhyMeasure/1 -> SensorOut/1

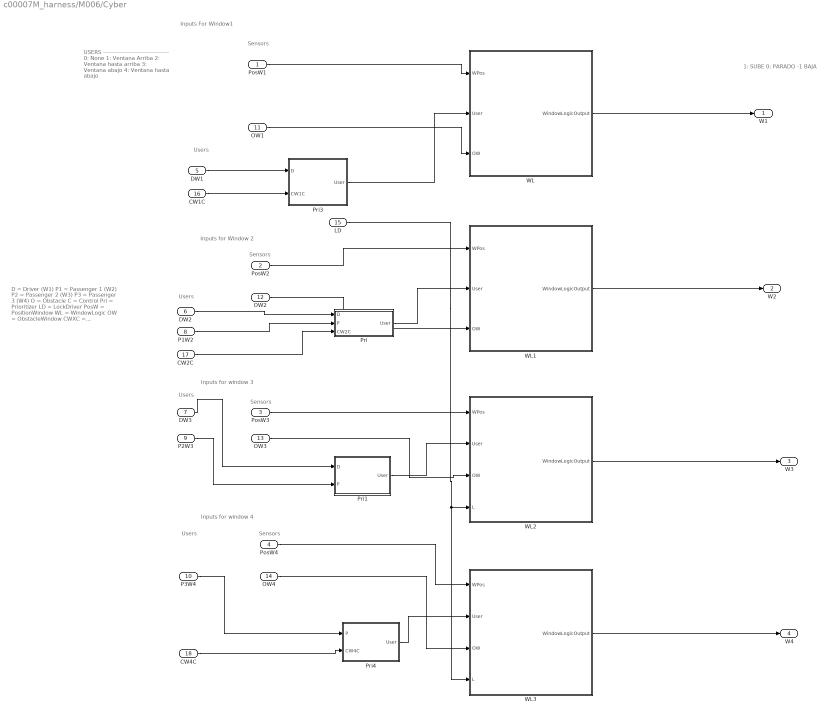
== system c00007M_harness/M006/Cyber ==
  note: Sensors
  note: Inputs For Window1
  note: Inputs for Window 2
  note: Inputs for window 3
  note: Inputs for window 4
  note: Users
  note: Users
  note: Sensors
  note: Users
  note: Sensors
  note: Users
  note: Sensors
  note: USERS
      | ---------------------------------
      | 0: None
      | 1: Ventana Arriba
      | 2: Ventana hasta arriba
      | 3: Ventana abajo
      | 4: Ventana hasta abajo
  note: 1: SUBE
      | 0: PARADO
      | -1 BAJA
  note: D = Driver (W1)
      | P1 = Passenger 1 (W2)
      | P2 = Passenger 2 (W3)
      | P3 = Passenger 3 (W4)
      | O = Obstacle
      | C = Control
      | Pri = Prioritizer
      | LD = LockDriver
      | PosW = PositionWindow
      | WL = WindowLogic
      | OW = ObstacleWindow
      | CWXC = ControlWindowXCentralized
      | S = Sensor
      | L = Lock
      | WPos = WindowPosition
      | M = Memory
      | InW = InputWindow
      | WIn = WindowInput
  PosW1 : Inport
  PosW2 : Inport  Port=2
  PosW3 : Inport  Port=3
  PosW4 : Inport  Port=4
  DW1 : Inport  Port=5
  DW2 : Inport  Port=6
  DW3 : Inport  Port=7
  P1W2 : Inport  Port=8
  P2W3 : Inport  Port=9
  P3W4 : Inport  Port=10
  OW1 : Inport  Port=11
  OW2 : Inport  Port=12
  OW3 : Inport  Port=13
  OW4 : Inport  Port=14
  LD : Inport  Port=15
  CW1C : Inport  Port=16
  CW2C : Inport  Port=17
  CW4C : Inport  Port=18
  Pri : Subsystem
  Pri1 : Subsystem
  Pri3 : Subsystem
  Pri4 : Subsystem
  WL : Subsystem
  WL1 : Subsystem
  WL2 : Subsystem
  WL3 : Subsystem
  W1 : Outport
  W2 : Outport  Port=2
  W3 : Outport  Port=3
  W4 : Outport  Port=4
  wires:
  CW4C/1 -> Pri4/2(CW4C)
  CW2C/1 -> Pri/3(CW2C)
  CW1C/1 -> Pri3/2(CW1C)
  Pri3/1(User) -> WL/2(User)
  WL3/1(WindowLogicOutput) -> W4/1
  WL2/1(WindowLogicOutput) -> W3/1
  Pri4/1(User) -> WL3/2(User)
  OW4/1 -> WL3/3(OW)
  PosW4/1 -> WL3/1(WPos)
  P3W4/1 -> Pri4/1(P)
  P2W3/1 -> Pri1/2(P)
  DW3/1 -> Pri1/1(D)
  OW3/1 -> WL2/3(OW)
  PosW3/1 -> WL2/1(WPos)
  Pri1/1(User) -> WL2/2(User)
  WL1/1(WindowLogicOutput) -> W2/1
  OW2/1 -> WL1/3(OW)
  PosW2/1 -> WL1/1(WPos)
  P1W2/1 -> Pri/2(P)
  DW2/1 -> Pri/1(D)
  Pri/1(User) -> WL1/2(User)
  WL/1(WindowLogicOutput) -> W1/1
  DW1/1 -> Pri3/1(D)
  OW1/1 -> WL/3(OW)
  PosW1/1 -> WL/1(WPos)
  LD/1 -> WL2/4(L), WL3/4(L)

== system c00007M_harness/M006/Physical ==
  InW1 : Inport
  InW2 : Inport  Port=2
  InW3 : Inport  Port=3
  InW4 : Inport  Port=4
  W : Subsystem
  W5 : Subsystem
  W6 : Subsystem
  W7 : Subsystem
  W1 : Outport
  W2 : Outport  Port=2
  W3 : Outport  Port=3
  W4 : Outport  Port=4
  wires:
  W7/1(WPos) -> W4/1
  W6/1(WPos) -> W3/1
  W5/1(WPos) -> W2/1
  W/1(WPos) -> W1/1
  InW4/1 -> W7/1(WIn)
  InW3/1 -> W6/1(WIn)
  InW2/1 -> W5/1(WIn)
  InW1/1 -> W/1(WIn)

== system c00007M_harness/M006/S1 ==
  PhyMeasure : Inport
  SensorOut : Outport
  wires:
  PhyMeasure/1 -> SensorOut/1

== system c00007M_harness/M006/S2 ==
  PhyMeasure : Inport
  SensorOut : Outport
  wires:
  PhyMeasure/1 -> SensorOut/1

== system c00007M_harness/M006/S3 ==
  PhyMeasure : Inport
  SensorOut : Outport
  wires:
  PhyMeasure/1 -> SensorOut/1

== system c00007M_harness/M006/S4 ==
  PhyMeasure : Inport
  SensorOut : Outport
  wires:
  PhyMeasure/1 -> SensorOut/1

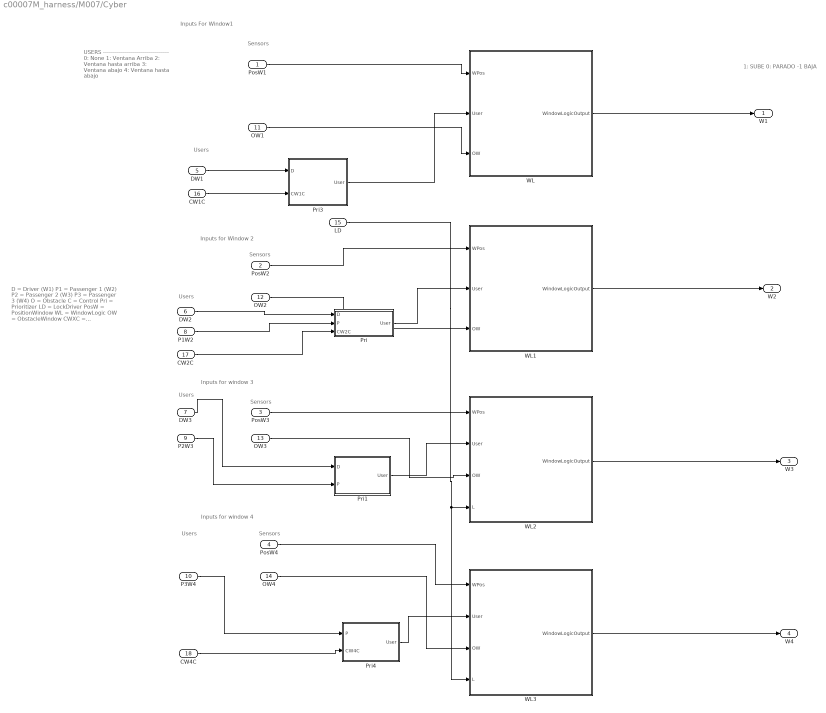
== system c00007M_harness/M007/Cyber ==
  note: Sensors
  note: Inputs For Window1
  note: Inputs for Window 2
  note: Inputs for window 3
  note: Inputs for window 4
  note: Users
  note: Users
  note: Sensors
  note: Users
  note: Sensors
  note: Users
  note: Sensors
  note: USERS
      | ---------------------------------
      | 0: None
      | 1: Ventana Arriba
      | 2: Ventana hasta arriba
      | 3: Ventana abajo
      | 4: Ventana hasta abajo
  note: 1: SUBE
      | 0: PARADO
      | -1 BAJA
  note: D = Driver (W1)
      | P1 = Passenger 1 (W2)
      | P2 = Passenger 2 (W3)
      | P3 = Passenger 3 (W4)
      | O = Obstacle
      | C = Control
      | Pri = Prioritizer
      | LD = LockDriver
      | PosW = PositionWindow
      | WL = WindowLogic
      | OW = ObstacleWindow
      | CWXC = ControlWindowXCentralized
      | S = Sensor
      | L = Lock
      | WPos = WindowPosition
      | M = Memory
      | InW = InputWindow
      | WIn = WindowInput
  PosW1 : Inport
  PosW2 : Inport  Port=2
  PosW3 : Inport  Port=3
  PosW4 : Inport  Port=4
  DW1 : Inport  Port=5
  DW2 : Inport  Port=6
  DW3 : Inport  Port=7
  P1W2 : Inport  Port=8
  P2W3 : Inport  Port=9
  P3W4 : Inport  Port=10
  OW1 : Inport  Port=11
  OW2 : Inport  Port=12
  OW3 : Inport  Port=13
  OW4 : Inport  Port=14
  LD : Inport  Port=15
  CW1C : Inport  Port=16
  CW2C : Inport  Port=17
  CW4C : Inport  Port=18
  Pri : Subsystem
  Pri1 : Subsystem
  Pri3 : Subsystem
  Pri4 : Subsystem
  WL : Subsystem
  WL1 : Subsystem
  WL2 : Subsystem
  WL3 : Subsystem
  W1 : Outport
  W2 : Outport  Port=2
  W3 : Outport  Port=3
  W4 : Outport  Port=4
  wires:
  CW4C/1 -> Pri4/2(CW4C)
  CW2C/1 -> Pri/3(CW2C)
  CW1C/1 -> Pri3/2(CW1C)
  Pri3/1(User) -> WL/2(User)
  WL3/1(WindowLogicOutput) -> W4/1
  WL2/1(WindowLogicOutput) -> W3/1
  Pri4/1(User) -> WL3/2(User)
  OW4/1 -> WL3/3(OW)
  PosW4/1 -> WL3/1(WPos)
  P3W4/1 -> Pri4/1(P)
  P2W3/1 -> Pri1/2(P)
  DW3/1 -> Pri1/1(D)
  OW3/1 -> WL2/3(OW)
  PosW3/1 -> WL2/1(WPos)
  Pri1/1(User) -> WL2/2(User)
  WL1/1(WindowLogicOutput) -> W2/1
  OW2/1 -> WL1/3(OW)
  PosW2/1 -> WL1/1(WPos)
  P1W2/1 -> Pri/2(P)
  DW2/1 -> Pri/1(D)
  Pri/1(User) -> WL1/2(User)
  WL/1(WindowLogicOutput) -> W1/1
  DW1/1 -> Pri3/1(D)
  OW1/1 -> WL/3(OW)
  PosW1/1 -> WL/1(WPos)
  LD/1 -> WL2/4(L), WL3/4(L)

== system c00007M_harness/M007/Physical ==
  InW1 : Inport
  InW2 : Inport  Port=2
  InW3 : Inport  Port=3
  InW4 : Inport  Port=4
  W : Subsystem
  W5 : Subsystem
  W6 : Subsystem
  W7 : Subsystem
  W1 : Outport
  W2 : Outport  Port=2
  W3 : Outport  Port=3
  W4 : Outport  Port=4
  wires:
  W7/1(WPos) -> W4/1
  W6/1(WPos) -> W3/1
  W5/1(WPos) -> W2/1
  W/1(WPos) -> W1/1
  InW4/1 -> W7/1(WIn)
  InW3/1 -> W6/1(WIn)
  InW2/1 -> W5/1(WIn)
  InW1/1 -> W/1(WIn)

== system c00007M_harness/M007/S1 ==
  PhyMeasure : Inport
  SensorOut : Outport
  wires:
  PhyMeasure/1 -> SensorOut/1

== system c00007M_harness/M007/S2 ==
  PhyMeasure : Inport
  SensorOut : Outport
  wires:
  PhyMeasure/1 -> SensorOut/1

== system c00007M_harness/M007/S3 ==
  PhyMeasure : Inport
  SensorOut : Outport
  wires:
  PhyMeasure/1 -> SensorOut/1

== system c00007M_harness/M007/S4 ==
  PhyMeasure : Inport
  SensorOut : Outport
  wires:
  PhyMeasure/1 -> SensorOut/1

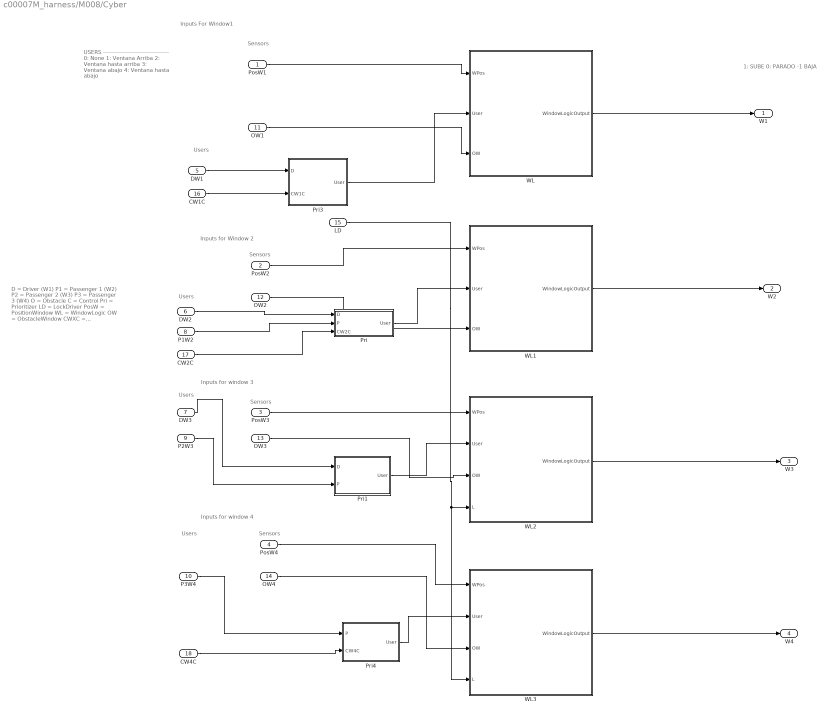
== system c00007M_harness/M008/Cyber ==
  note: Sensors
  note: Inputs For Window1
  note: Inputs for Window 2
  note: Inputs for window 3
  note: Inputs for window 4
  note: Users
  note: Users
  note: Sensors
  note: Users
  note: Sensors
  note: Users
  note: Sensors
  note: USERS
      | ---------------------------------
      | 0: None
      | 1: Ventana Arriba
      | 2: Ventana hasta arriba
      | 3: Ventana abajo
      | 4: Ventana hasta abajo
  note: 1: SUBE
      | 0: PARADO
      | -1 BAJA
  note: D = Driver (W1)
      | P1 = Passenger 1 (W2)
      | P2 = Passenger 2 (W3)
      | P3 = Passenger 3 (W4)
      | O = Obstacle
      | C = Control
      | Pri = Prioritizer
      | LD = LockDriver
      | PosW = PositionWindow
      | WL = WindowLogic
      | OW = ObstacleWindow
      | CWXC = ControlWindowXCentralized
      | S = Sensor
      | L = Lock
      | WPos = WindowPosition
      | M = Memory
      | InW = InputWindow
      | WIn = WindowInput
  PosW1 : Inport
  PosW2 : Inport  Port=2
  PosW3 : Inport  Port=3
  PosW4 : Inport  Port=4
  DW1 : Inport  Port=5
  DW2 : Inport  Port=6
  DW3 : Inport  Port=7
  P1W2 : Inport  Port=8
  P2W3 : Inport  Port=9
  P3W4 : Inport  Port=10
  OW1 : Inport  Port=11
  OW2 : Inport  Port=12
  OW3 : Inport  Port=13
  OW4 : Inport  Port=14
  LD : Inport  Port=15
  CW1C : Inport  Port=16
  CW2C : Inport  Port=17
  CW4C : Inport  Port=18
  Pri : Subsystem
  Pri1 : Subsystem
  Pri3 : Subsystem
  Pri4 : Subsystem
  WL : Subsystem
  WL1 : Subsystem
  WL2 : Subsystem
  WL3 : Subsystem
  W1 : Outport
  W2 : Outport  Port=2
  W3 : Outport  Port=3
  W4 : Outport  Port=4
  wires:
  CW4C/1 -> Pri4/2(CW4C)
  CW2C/1 -> Pri/3(CW2C)
  CW1C/1 -> Pri3/2(CW1C)
  Pri3/1(User) -> WL/2(User)
  WL3/1(WindowLogicOutput) -> W4/1
  WL2/1(WindowLogicOutput) -> W3/1
  Pri4/1(User) -> WL3/2(User)
  OW4/1 -> WL3/3(OW)
  PosW4/1 -> WL3/1(WPos)
  P3W4/1 -> Pri4/1(P)
  P2W3/1 -> Pri1/2(P)
  DW3/1 -> Pri1/1(D)
  OW3/1 -> WL2/3(OW)
  PosW3/1 -> WL2/1(WPos)
  Pri1/1(User) -> WL2/2(User)
  WL1/1(WindowLogicOutput) -> W2/1
  OW2/1 -> WL1/3(OW)
  PosW2/1 -> WL1/1(WPos)
  P1W2/1 -> Pri/2(P)
  DW2/1 -> Pri/1(D)
  Pri/1(User) -> WL1/2(User)
  WL/1(WindowLogicOutput) -> W1/1
  DW1/1 -> Pri3/1(D)
  OW1/1 -> WL/3(OW)
  PosW1/1 -> WL/1(WPos)
  LD/1 -> WL2/4(L), WL3/4(L)

== system c00007M_harness/M008/Physical ==
  InW1 : Inport
  InW2 : Inport  Port=2
  InW3 : Inport  Port=3
  InW4 : Inport  Port=4
  W : Subsystem
  W5 : Subsystem
  W6 : Subsystem
  W7 : Subsystem
  W1 : Outport
  W2 : Outport  Port=2
  W3 : Outport  Port=3
  W4 : Outport  Port=4
  wires:
  W7/1(WPos) -> W4/1
  W6/1(WPos) -> W3/1
  W5/1(WPos) -> W2/1
  W/1(WPos) -> W1/1
  InW4/1 -> W7/1(WIn)
  InW3/1 -> W6/1(WIn)
  InW2/1 -> W5/1(WIn)
  InW1/1 -> W/1(WIn)

== system c00007M_harness/M008/S1 ==
  PhyMeasure : Inport
  SensorOut : Outport
  wires:
  PhyMeasure/1 -> SensorOut/1

== system c00007M_harness/M008/S2 ==
  PhyMeasure : Inport
  SensorOut : Outport
  wires:
  PhyMeasure/1 -> SensorOut/1

== system c00007M_harness/M008/S3 ==
  PhyMeasure : Inport
  SensorOut : Outport
  wires:
  PhyMeasure/1 -> SensorOut/1

== system c00007M_harness/M008/S4 ==
  PhyMeasure : Inport
  SensorOut : Outport
  wires:
  PhyMeasure/1 -> SensorOut/1

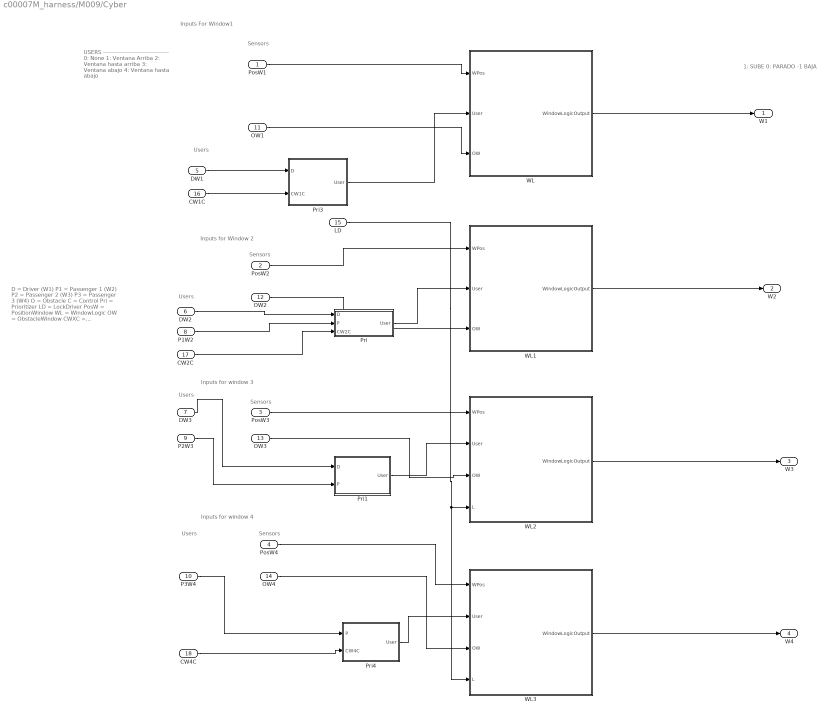
== system c00007M_harness/M009/Cyber ==
  note: Sensors
  note: Inputs For Window1
  note: Inputs for Window 2
  note: Inputs for window 3
  note: Inputs for window 4
  note: Users
  note: Users
  note: Sensors
  note: Users
  note: Sensors
  note: Users
  note: Sensors
  note: USERS
      | ---------------------------------
      | 0: None
      | 1: Ventana Arriba
      | 2: Ventana hasta arriba
      | 3: Ventana abajo
      | 4: Ventana hasta abajo
  note: 1: SUBE
      | 0: PARADO
      | -1 BAJA
  note: D = Driver (W1)
      | P1 = Passenger 1 (W2)
      | P2 = Passenger 2 (W3)
      | P3 = Passenger 3 (W4)
      | O = Obstacle
      | C = Control
      | Pri = Prioritizer
      | LD = LockDriver
      | PosW = PositionWindow
      | WL = WindowLogic
      | OW = ObstacleWindow
      | CWXC = ControlWindowXCentralized
      | S = Sensor
      | L = Lock
      | WPos = WindowPosition
      | M = Memory
      | InW = InputWindow
      | WIn = WindowInput
  PosW1 : Inport
  PosW2 : Inport  Port=2
  PosW3 : Inport  Port=3
  PosW4 : Inport  Port=4
  DW1 : Inport  Port=5
  DW2 : Inport  Port=6
  DW3 : Inport  Port=7
  P1W2 : Inport  Port=8
  P2W3 : Inport  Port=9
  P3W4 : Inport  Port=10
  OW1 : Inport  Port=11
  OW2 : Inport  Port=12
  OW3 : Inport  Port=13
  OW4 : Inport  Port=14
  LD : Inport  Port=15
  CW1C : Inport  Port=16
  CW2C : Inport  Port=17
  CW4C : Inport  Port=18
  Pri : Subsystem
  Pri1 : Subsystem
  Pri3 : Subsystem
  Pri4 : Subsystem
  WL : Subsystem
  WL1 : Subsystem
  WL2 : Subsystem
  WL3 : Subsystem
  W1 : Outport
  W2 : Outport  Port=2
  W3 : Outport  Port=3
  W4 : Outport  Port=4
  wires:
  CW4C/1 -> Pri4/2(CW4C)
  CW2C/1 -> Pri/3(CW2C)
  CW1C/1 -> Pri3/2(CW1C)
  Pri3/1(User) -> WL/2(User)
  WL3/1(WindowLogicOutput) -> W4/1
  WL2/1(WindowLogicOutput) -> W3/1
  Pri4/1(User) -> WL3/2(User)
  OW4/1 -> WL3/3(OW)
  PosW4/1 -> WL3/1(WPos)
  P3W4/1 -> Pri4/1(P)
  P2W3/1 -> Pri1/2(P)
  DW3/1 -> Pri1/1(D)
  OW3/1 -> WL2/3(OW)
  PosW3/1 -> WL2/1(WPos)
  Pri1/1(User) -> WL2/2(User)
  WL1/1(WindowLogicOutput) -> W2/1
  OW2/1 -> WL1/3(OW)
  PosW2/1 -> WL1/1(WPos)
  P1W2/1 -> Pri/2(P)
  DW2/1 -> Pri/1(D)
  Pri/1(User) -> WL1/2(User)
  WL/1(WindowLogicOutput) -> W1/1
  DW1/1 -> Pri3/1(D)
  OW1/1 -> WL/3(OW)
  PosW1/1 -> WL/1(WPos)
  LD/1 -> WL2/4(L), WL3/4(L)

== system c00007M_harness/M009/Physical ==
  InW1 : Inport
  InW2 : Inport  Port=2
  InW3 : Inport  Port=3
  InW4 : Inport  Port=4
  W : Subsystem
  W5 : Subsystem
  W6 : Subsystem
  W7 : Subsystem
  W1 : Outport
  W2 : Outport  Port=2
  W3 : Outport  Port=3
  W4 : Outport  Port=4
  wires:
  W7/1(WPos) -> W4/1
  W6/1(WPos) -> W3/1
  W5/1(WPos) -> W2/1
  W/1(WPos) -> W1/1
  InW4/1 -> W7/1(WIn)
  InW3/1 -> W6/1(WIn)
  InW2/1 -> W5/1(WIn)
  InW1/1 -> W/1(WIn)

== system c00007M_harness/M009/S1 ==
  PhyMeasure : Inport
  SensorOut : Outport
  wires:
  PhyMeasure/1 -> SensorOut/1

== system c00007M_harness/M009/S2 ==
  PhyMeasure : Inport
  SensorOut : Outport
  wires:
  PhyMeasure/1 -> SensorOut/1

== system c00007M_harness/M009/S3 ==
  PhyMeasure : Inport
  SensorOut : Outport
  wires:
  PhyMeasure/1 -> SensorOut/1

== system c00007M_harness/M009/S4 ==
  PhyMeasure : Inport
  SensorOut : Outport
  wires:
  PhyMeasure/1 -> SensorOut/1

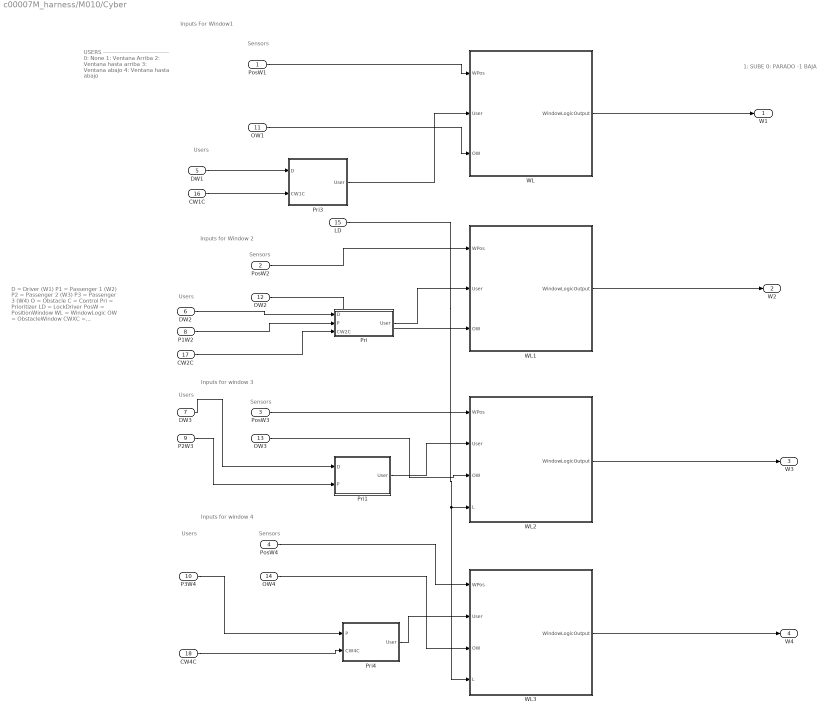
== system c00007M_harness/M010/Cyber ==
  note: Sensors
  note: Inputs For Window1
  note: Inputs for Window 2
  note: Inputs for window 3
  note: Inputs for window 4
  note: Users
  note: Users
  note: Sensors
  note: Users
  note: Sensors
  note: Users
  note: Sensors
  note: USERS
      | ---------------------------------
      | 0: None
      | 1: Ventana Arriba
      | 2: Ventana hasta arriba
      | 3: Ventana abajo
      | 4: Ventana hasta abajo
  note: 1: SUBE
      | 0: PARADO
      | -1 BAJA
  note: D = Driver (W1)
      | P1 = Passenger 1 (W2)
      | P2 = Passenger 2 (W3)
      | P3 = Passenger 3 (W4)
      | O = Obstacle
      | C = Control
      | Pri = Prioritizer
      | LD = LockDriver
      | PosW = PositionWindow
      | WL = WindowLogic
      | OW = ObstacleWindow
      | CWXC = ControlWindowXCentralized
      | S = Sensor
      | L = Lock
      | WPos = WindowPosition
      | M = Memory
      | InW = InputWindow
      | WIn = WindowInput
  PosW1 : Inport
  PosW2 : Inport  Port=2
  PosW3 : Inport  Port=3
  PosW4 : Inport  Port=4
  DW1 : Inport  Port=5
  DW2 : Inport  Port=6
  DW3 : Inport  Port=7
  P1W2 : Inport  Port=8
  P2W3 : Inport  Port=9
  P3W4 : Inport  Port=10
  OW1 : Inport  Port=11
  OW2 : Inport  Port=12
  OW3 : Inport  Port=13
  OW4 : Inport  Port=14
  LD : Inport  Port=15
  CW1C : Inport  Port=16
  CW2C : Inport  Port=17
  CW4C : Inport  Port=18
  Pri : Subsystem
  Pri1 : Subsystem
  Pri3 : Subsystem
  Pri4 : Subsystem
  WL : Subsystem
  WL1 : Subsystem
  WL2 : Subsystem
  WL3 : Subsystem
  W1 : Outport
  W2 : Outport  Port=2
  W3 : Outport  Port=3
  W4 : Outport  Port=4
  wires:
  CW4C/1 -> Pri4/2(CW4C)
  CW2C/1 -> Pri/3(CW2C)
  CW1C/1 -> Pri3/2(CW1C)
  Pri3/1(User) -> WL/2(User)
  WL3/1(WindowLogicOutput) -> W4/1
  WL2/1(WindowLogicOutput) -> W3/1
  Pri4/1(User) -> WL3/2(User)
  OW4/1 -> WL3/3(OW)
  PosW4/1 -> WL3/1(WPos)
  P3W4/1 -> Pri4/1(P)
  P2W3/1 -> Pri1/2(P)
  DW3/1 -> Pri1/1(D)
  OW3/1 -> WL2/3(OW)
  PosW3/1 -> WL2/1(WPos)
  Pri1/1(User) -> WL2/2(User)
  WL1/1(WindowLogicOutput) -> W2/1
  OW2/1 -> WL1/3(OW)
  PosW2/1 -> WL1/1(WPos)
  P1W2/1 -> Pri/2(P)
  DW2/1 -> Pri/1(D)
  Pri/1(User) -> WL1/2(User)
  WL/1(WindowLogicOutput) -> W1/1
  DW1/1 -> Pri3/1(D)
  OW1/1 -> WL/3(OW)
  PosW1/1 -> WL/1(WPos)
  LD/1 -> WL2/4(L), WL3/4(L)

== system c00007M_harness/M010/Physical ==
  InW1 : Inport
  InW2 : Inport  Port=2
  InW3 : Inport  Port=3
  InW4 : Inport  Port=4
  W : Subsystem
  W5 : Subsystem
  W6 : Subsystem
  W7 : Subsystem
  W1 : Outport
  W2 : Outport  Port=2
  W3 : Outport  Port=3
  W4 : Outport  Port=4
  wires:
  W7/1(WPos) -> W4/1
  W6/1(WPos) -> W3/1
  W5/1(WPos) -> W2/1
  W/1(WPos) -> W1/1
  InW4/1 -> W7/1(WIn)
  InW3/1 -> W6/1(WIn)
  InW2/1 -> W5/1(WIn)
  InW1/1 -> W/1(WIn)

== system c00007M_harness/M010/S1 ==
  PhyMeasure : Inport
  SensorOut : Outport
  wires:
  PhyMeasure/1 -> SensorOut/1

== system c00007M_harness/M010/S2 ==
  PhyMeasure : Inport
  SensorOut : Outport
  wires:
  PhyMeasure/1 -> SensorOut/1

== system c00007M_harness/M010/S3 ==
  PhyMeasure : Inport
  SensorOut : Outport
  wires:
  PhyMeasure/1 -> SensorOut/1

== system c00007M_harness/M010/S4 ==
  PhyMeasure : Inport
  SensorOut : Outport
  wires:
  PhyMeasure/1 -> SensorOut/1

== system c00007M_harness/M011/Cyber ==
  note: Sensors
  note: Inputs For Window1
  note: Inputs for Window 2
  note: Inputs for window 3
  note: Inputs for window 4
  note: Users
  note: Users
  note: Sensors
  note: Users
  note: Sensors
  note: Users
  note: Sensors
  note: USERS
      | ---------------------------------
      | 0: None
      | 1: Ventana Arriba
      | 2: Ventana hasta arriba
      | 3: Ventana abajo
      | 4: Ventana hasta abajo
  note: 1: SUBE
      | 0: PARADO
      | -1 BAJA
  note: D = Driver (W1)
      | P1 = Passenger 1 (W2)
      | P2 = Passenger 2 (W3)
      | P3 = Passenger 3 (W4)
      | O = Obstacle
      | C = Control
      | Pri = Prioritizer
      | LD = LockDriver
      | PosW = PositionWindow
      | WL = WindowLogic
      | OW = ObstacleWindow
      | CWXC = ControlWindowXCentralized
      | S = Sensor
      | L = Lock
      | WPos = WindowPosition
      | M = Memory
      | InW = InputWindow
      | WIn = WindowInput
  PosW1 : Inport
  PosW2 : Inport  Port=2
  PosW3 : Inport  Port=3
  PosW4 : Inport  Port=4
  DW1 : Inport  Port=5
  DW2 : Inport  Port=6
  DW3 : Inport  Port=7
  P1W2 : Inport  Port=8
  P2W3 : Inport  Port=9
  P3W4 : Inport  Port=10
  OW1 : Inport  Port=11
  OW2 : Inport  Port=12
  OW3 : Inport  Port=13
  OW4 : Inport  Port=14
  LD : Inport  Port=15
  CW1C : Inport  Port=16
  CW2C : Inport  Port=17
  CW4C : Inport  Port=18
  Pri : Subsystem
  Pri1 : Subsystem
  Pri3 : Subsystem
  Pri4 : Subsystem
  WL : Subsystem
  WL1 : Subsystem
  WL2 : Subsystem
  WL3 : Subsystem
  W1 : Outport
  W2 : Outport  Port=2
  W3 : Outport  Port=3
  W4 : Outport  Port=4
  wires:
  CW4C/1 -> Pri4/2(CW4C)
  CW2C/1 -> Pri/3(CW2C)
  CW1C/1 -> Pri3/2(CW1C)
  Pri3/1(User) -> WL/2(User)
  WL3/1(WindowLogicOutput) -> W4/1
  WL2/1(WindowLogicOutput) -> W3/1
  Pri4/1(User) -> WL3/2(User)
  OW4/1 -> WL3/3(OW)
  PosW4/1 -> WL3/1(WPos)
  P3W4/1 -> Pri4/1(P)
  P2W3/1 -> Pri1/2(P)
  DW3/1 -> Pri1/1(D)
  OW3/1 -> WL2/3(OW)
  PosW3/1 -> WL2/1(WPos)
  Pri1/1(User) -> WL2/2(User)
  WL1/1(WindowLogicOutput) -> W2/1
  OW2/1 -> WL1/3(OW)
  PosW2/1 -> WL1/1(WPos)
  P1W2/1 -> Pri/2(P)
  DW2/1 -> Pri/1(D)
  Pri/1(User) -> WL1/2(User)
  WL/1(WindowLogicOutput) -> W1/1
  DW1/1 -> Pri3/1(D)
  OW1/1 -> WL/3(OW)
  PosW1/1 -> WL/1(WPos)
  LD/1 -> WL2/4(L), WL3/4(L)

== system c00007M_harness/M011/Physical ==
  InW1 : Inport
  InW2 : Inport  Port=2
  InW3 : Inport  Port=3
  InW4 : Inport  Port=4
  W : Subsystem
  W5 : Subsystem
  W6 : Subsystem
  W7 : Subsystem
  W1 : Outport
  W2 : Outport  Port=2
  W3 : Outport  Port=3
  W4 : Outport  Port=4
  wires:
  W7/1(WPos) -> W4/1
  W6/1(WPos) -> W3/1
  W5/1(WPos) -> W2/1
  W/1(WPos) -> W1/1
  InW4/1 -> W7/1(WIn)
  InW3/1 -> W6/1(WIn)
  InW2/1 -> W5/1(WIn)
  InW1/1 -> W/1(WIn)

== system c00007M_harness/M011/S1 ==
  PhyMeasure : Inport
  Add : Sum
  Constant : Constant
  SensorOut : Outport
  wires:
  PhyMeasure/1 -> Add/2
  Add/1 -> SensorOut/1
  Constant/1 -> Add/1

== system c00007M_harness/M011/S2 ==
  PhyMeasure : Inport
  SensorOut : Outport
  wires:
  PhyMeasure/1 -> SensorOut/1

== system c00007M_harness/M011/S3 ==
  PhyMeasure : Inport
  SensorOut : Outport
  wires:
  PhyMeasure/1 -> SensorOut/1

== system c00007M_harness/M011/S4 ==
  PhyMeasure : Inport
  SensorOut : Outport
  wires:
  PhyMeasure/1 -> SensorOut/1

== system c00007M_harness/M012/Cyber ==
  note: Sensors
  note: Inputs For Window1
  note: Inputs for Window 2
  note: Inputs for window 3
  note: Inputs for window 4
  note: Users
  note: Users
  note: Sensors
  note: Users
  note: Sensors
  note: Users
  note: Sensors
  note: USERS
      | ---------------------------------
      | 0: None
      | 1: Ventana Arriba
      | 2: Ventana hasta arriba
      | 3: Ventana abajo
      | 4: Ventana hasta abajo
  note: 1: SUBE
      | 0: PARADO
      | -1 BAJA
  note: D = Driver (W1)
      | P1 = Passenger 1 (W2)
      | P2 = Passenger 2 (W3)
      | P3 = Passenger 3 (W4)
      | O = Obstacle
      | C = Control
      | Pri = Prioritizer
      | LD = LockDriver
      | PosW = PositionWindow
      | WL = WindowLogic
      | OW = ObstacleWindow
      | CWXC = ControlWindowXCentralized
      | S = Sensor
      | L = Lock
      | WPos = WindowPosition
      | M = Memory
      | InW = InputWindow
      | WIn = WindowInput
  PosW1 : Inport
  PosW2 : Inport  Port=2
  PosW3 : Inport  Port=3
  PosW4 : Inport  Port=4
  DW1 : Inport  Port=5
  DW2 : Inport  Port=6
  DW3 : Inport  Port=7
  P1W2 : Inport  Port=8
  P2W3 : Inport  Port=9
  P3W4 : Inport  Port=10
  OW1 : Inport  Port=11
  OW2 : Inport  Port=12
  OW3 : Inport  Port=13
  OW4 : Inport  Port=14
  LD : Inport  Port=15
  CW1C : Inport  Port=16
  CW2C : Inport  Port=17
  CW4C : Inport  Port=18
  Pri : Subsystem
  Pri1 : Subsystem
  Pri3 : Subsystem
  Pri4 : Subsystem
  WL : Subsystem
  WL1 : Subsystem
  WL2 : Subsystem
  WL3 : Subsystem
  W1 : Outport
  W2 : Outport  Port=2
  W3 : Outport  Port=3
  W4 : Outport  Port=4
  wires:
  CW4C/1 -> Pri4/2(CW4C)
  CW2C/1 -> Pri/3(CW2C)
  CW1C/1 -> Pri3/2(CW1C)
  Pri3/1(User) -> WL/2(User)
  WL3/1(WindowLogicOutput) -> W4/1
  WL2/1(WindowLogicOutput) -> W3/1
  Pri4/1(User) -> WL3/2(User)
  OW4/1 -> WL3/3(OW)
  PosW4/1 -> WL3/1(WPos)
  P3W4/1 -> Pri4/1(P)
  P2W3/1 -> Pri1/2(P)
  DW3/1 -> Pri1/1(D)
  OW3/1 -> WL2/3(OW)
  PosW3/1 -> WL2/1(WPos)
  Pri1/1(User) -> WL2/2(User)
  WL1/1(WindowLogicOutput) -> W2/1
  OW2/1 -> WL1/3(OW)
  PosW2/1 -> WL1/1(WPos)
  P1W2/1 -> Pri/2(P)
  DW2/1 -> Pri/1(D)
  Pri/1(User) -> WL1/2(User)
  WL/1(WindowLogicOutput) -> W1/1
  DW1/1 -> Pri3/1(D)
  OW1/1 -> WL/3(OW)
  PosW1/1 -> WL/1(WPos)
  LD/1 -> WL2/4(L), WL3/4(L)

== system c00007M_harness/M012/Physical ==
  InW1 : Inport
  InW2 : Inport  Port=2
  InW3 : Inport  Port=3
  InW4 : Inport  Port=4
  W : Subsystem
  W5 : Subsystem
  W6 : Subsystem
  W7 : Subsystem
  W1 : Outport
  W2 : Outport  Port=2
  W3 : Outport  Port=3
  W4 : Outport  Port=4
  wires:
  W7/1(WPos) -> W4/1
  W6/1(WPos) -> W3/1
  W5/1(WPos) -> W2/1
  W/1(WPos) -> W1/1
  InW4/1 -> W7/1(WIn)
  InW3/1 -> W6/1(WIn)
  InW2/1 -> W5/1(WIn)
  InW1/1 -> W/1(WIn)

== system c00007M_harness/M012/S1 ==
  PhyMeasure : Inport
  SensorOut : Outport
  wires:
  PhyMeasure/1 -> SensorOut/1

== system c00007M_harness/M012/S2 ==
  PhyMeasure : Inport
  Add : Sum
  Constant : Constant
  SensorOut : Outport
  wires:
  PhyMeasure/1 -> Add/2
  Constant/1 -> Add/1
  Add/1 -> SensorOut/1

== system c00007M_harness/M012/S3 ==
  PhyMeasure : Inport
  SensorOut : Outport
  wires:
  PhyMeasure/1 -> SensorOut/1

== system c00007M_harness/M012/S4 ==
  PhyMeasure : Inport
  SensorOut : Outport
  wires:
  PhyMeasure/1 -> SensorOut/1
